simulink model "s3EM"  (R2026b)
settings: Solver=VariableStepAuto
undefined symbols (not defined in the file): PlntEMMass
libraries: autolibsharedcommon x1
settings Model: ModifiedByFormat=The MathWorks, Inc.  Creator=The MathWorks, Inc.  LastModifiedBy=The MathWorks, Inc.

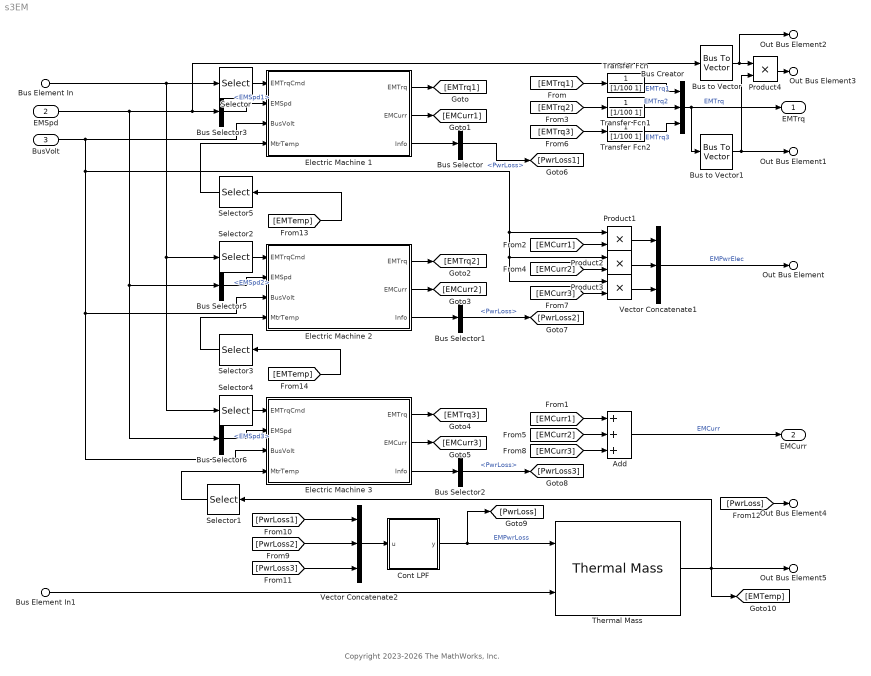
== system s3EM ==
  note: Copyright 2023-2026 The MathWorks, Inc.
  Bus Element In : Inport  PortName=Cntrl  Element=Vcu.EMTrqCmd
  EMSpd : Inport  Port=2
  BusVolt : Inport  Port=3
  Bus Element In1 : Inport  Port=4  PortName=Thermal  Element=Qem
  Add : Sum  Inputs=+++
  Bus Creator : BusCreator  Inputs=3
  Bus Selector : BusSelector  OutputSignals=PwrLoss
  Bus Selector1 : BusSelector  OutputSignals=PwrLoss
  Bus Selector2 : BusSelector  OutputSignals=PwrLoss
  Bus Selector3 : BusSelector  OutputSignals=EMSpd1
  Bus Selector5 : BusSelector  OutputSignals=EMSpd2
  Bus Selector6 : BusSelector  OutputSignals=EMSpd3
  Bus to Vector : BusToVector
  Bus to Vector1 : BusToVector
  Cont LPF : Subsystem
  Electric Machine 1 : Subsystem  Variant=on  VariantControlMode=label  LabelModeActiveChoice=Mapped EM
  Electric Machine 2 : Subsystem  Variant=on  VariantControlMode=label  LabelModeActiveChoice=Mapped EM
  Electric Machine 3 : Subsystem  Variant=on  VariantControlMode=label  LabelModeActiveChoice=Mapped EM
  Product{1..4} (4 alike) : Product
  Selector : Selector  InputPortWidth=3  IndexOptions=Index vector (dialog)  Indices=[1]  OutputSizes=1
  Selector1 : Selector  InputPortWidth=3  IndexOptions=Index vector (dialog)  Indices=[3]  OutputSizes=1
  Selector2 : Selector  InputPortWidth=3  IndexOptions=Index vector (dialog)  Indices=[2]  OutputSizes=1
  Selector3 : Selector  InputPortWidth=3  IndexOptions=Index vector (dialog)  Indices=[2]  OutputSizes=1
  Selector4 : Selector  InputPortWidth=3  IndexOptions=Index vector (dialog)  Indices=[3]  OutputSizes=1
  Selector5 : Selector  InputPortWidth=3  IndexOptions=Index vector (dialog)  Indices=[1]  OutputSizes=1
  Thermal Mass : autolibsharedcommon/Thermal Mass  Mass=PlntEMMass*ones(1,3)  Cp=PlntEMCp
  Transfer Fcn : TransferFcn  Denominator=[1/100 1]
  Transfer Fcn1 : TransferFcn  Denominator=[1/100 1]
  Transfer Fcn2 : TransferFcn  Denominator=[1/100 1]
  Vector Concatenate1 : Concatenate  NumInputs=3
  Vector Concatenate2 : Concatenate  NumInputs=3
  EMTrq : Outport
  EMCurr : Outport  Port=2
  Out Bus Element : Outport  Port=3  PortName=EMInfo  Element=EMPwrElec
  Out Bus Element1 : Outport  Port=3  PortName=EMInfo  Element=EMTrq
  Out Bus Element2 : Outport  Port=3  PortName=EMInfo  Element=EMSpd
  Out Bus Element3 : Outport  Port=3  PortName=EMInfo  Element=EMMechPwr
  Out Bus Element4 : Outport  Port=3  PortName=EMInfo  Element=EMPwrLoss
  Out Bus Element5 : Outport  Port=3  PortName=EMInfo  Element=EMTemp
  wires:
  Product3/1 -> Vector Concatenate1/3
  [EMCurr3] -> Product3/2
  [EMCurr3] -> Add/3
  Electric Machine 3/2(EMCurr) -> [EMCurr3]
  Electric Machine 3/1(EMTrq) -> [EMTrq3]
  Selector4/1 -> Electric Machine 3/1(EMTrqCmd)
  Bus Creator/1 -> Bus to Vector1/1, EMTrq/1  "EMTrq"
  BusVolt/1 -> Electric Machine 1/3(BusVolt), Electric Machine 3/3(BusVolt), Electric Machine 2/3(BusVolt), Product1/1, Product3/1, Product2/1
  Vector Concatenate1/1 -> Out Bus Element/1  "EMPwrElec"
  Bus Selector3/1 -> Electric Machine 1/2(EMSpd)  "<EMSpd1>"
  Bus Selector5/1 -> Electric Machine 2/2(EMSpd)  "<EMSpd2>"
  Bus Element In/1 -> Selector/1, Selector2/1, Selector4/1
  Product1/1 -> Vector Concatenate1/1
  Product2/1 -> Vector Concatenate1/2
  Selector2/1 -> Electric Machine 2/1(EMTrqCmd)
  Add/1 -> EMCurr/1  "EMCurr"
  Selector/1 -> Electric Machine 1/1(EMTrqCmd)
  Electric Machine 1/1(EMTrq) -> [EMTrq1]
  Electric Machine 1/2(EMCurr) -> [EMCurr1]
  [EMCurr1] -> Add/1
  [EMCurr1] -> Product1/2
  [EMCurr2] -> Product2/2
  [EMCurr2] -> Add/2
  Electric Machine 2/1(EMTrq) -> [EMTrq2]
  Electric Machine 2/2(EMCurr) -> [EMCurr2]
  Electric Machine 1/3(Info) -> Bus Selector/1
  Electric Machine 2/3(Info) -> Bus Selector1/1
  Electric Machine 3/3(Info) -> Bus Selector2/1
  Bus Selector/1 -> [PwrLoss1]  "<PwrLoss>"
  Bus Selector1/1 -> [PwrLoss2]  "<PwrLoss>"
  Bus Selector2/1 -> [PwrLoss3]  "<PwrLoss>"
  [PwrLoss1] -> Vector Concatenate2/1
  [PwrLoss2] -> Vector Concatenate2/2
  [PwrLoss3] -> Vector Concatenate2/3
  Vector Concatenate2/1 -> Cont LPF/1(u)
  Cont LPF/1(y) -> [PwrLoss], Thermal Mass/1  "EMPwrLoss"
  Thermal Mass/1 -> [EMTemp], Out Bus Element5/1, Selector1/1
  Product4/1 -> Out Bus Element3/1
  EMSpd/1 -> Bus to Vector/1, Bus Selector3/1, Bus Selector5/1, Bus Selector6/1
  Bus to Vector/1 -> Out Bus Element2/1, Product4/1
  Bus to Vector1/1 -> Out Bus Element1/1, Product4/2
  Bus Selector6/1 -> Electric Machine 3/2(EMSpd)  "<EMSpd3>"
  Selector1/1 -> Electric Machine 3/4(MtrTemp)
  Selector3/1 -> Electric Machine 2/4(MtrTemp)
  Selector5/1 -> Electric Machine 1/4(MtrTemp)
  Bus Element In1/1 -> Thermal Mass/2
  [PwrLoss] -> Out Bus Element4/1
  [EMTemp] -> Selector5/1
  [EMTemp] -> Selector3/1
  Transfer Fcn/1 -> Bus Creator/1  "EMTrq1"
  Transfer Fcn2/1 -> Bus Creator/3  "EMTrq3"
  Transfer Fcn1/1 -> Bus Creator/2  "EMTrq2"
  [EMTrq1] -> Transfer Fcn/1
  [EMTrq2] -> Transfer Fcn1/1
  [EMTrq3] -> Transfer Fcn2/1

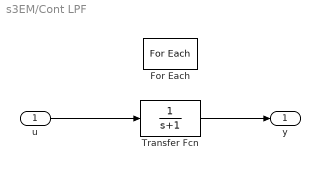
== system s3EM/Cont LPF ==
  u : Inport  Partition=on  PartitionDimension=1  PartitionWidth=1  PartitionOffset=0
  For Each : ForEach  DisableCoverage=on
  Transfer Fcn : TransferFcn  Denominator=[1 1]
  y : Outport  ConcatenationDimension=1
  wires:
  u/1 -> Transfer Fcn/1
  Transfer Fcn/1 -> y/1

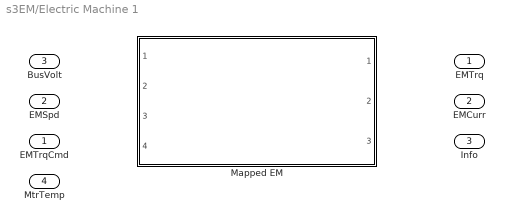
== system s3EM/Electric Machine 1 ==
  EMTrqCmd : Inport
  EMSpd : Inport  Port=2
  BusVolt : Inport  Port=3
  MtrTemp : Inport  Port=4
  Mapped EM : Subsystem  VariantControl=Mapped EM  ReferencedSubsystem=ElectricMachine1
  EMTrq : Outport  VectorParamsAs1DForOutWhenUnconnected=off
  EMCurr : Outport  Port=2  VectorParamsAs1DForOutWhenUnconnected=off
  Info : Outport  Port=3

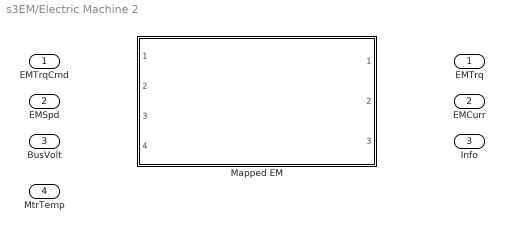
== system s3EM/Electric Machine 2 ==
  EMTrqCmd : Inport
  EMSpd : Inport  Port=2
  BusVolt : Inport  Port=3
  MtrTemp : Inport  Port=4
  Mapped EM : Subsystem  VariantControl=Mapped EM  ReferencedSubsystem=ElectricMachine2
  EMTrq : Outport  VectorParamsAs1DForOutWhenUnconnected=off
  EMCurr : Outport  Port=2  VectorParamsAs1DForOutWhenUnconnected=off
  Info : Outport  Port=3

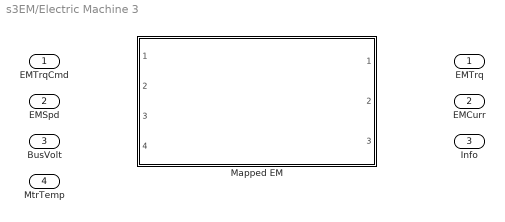
== system s3EM/Electric Machine 3 ==
  EMTrqCmd : Inport
  EMSpd : Inport  Port=2
  BusVolt : Inport  Port=3
  MtrTemp : Inport  Port=4
  Mapped EM : Subsystem  VariantControl=Mapped EM  ReferencedSubsystem=ElectricMachine3
  EMTrq : Outport  VectorParamsAs1DForOutWhenUnconnected=off
  EMCurr : Outport  Port=2  VectorParamsAs1DForOutWhenUnconnected=off
  Info : Outport  Port=3
